simulink model "distillation"  (R2013a)
settings: Solver=ode45  StartTime=0.0  StopTime=100  RelTol=1e-3
StopFcn:
  | plot_results
libraries: simulink x4, realtime_pacer_lib x1
settings Model: Creator=tsladeche  LastModifiedBy=John
settings DataIOCC: SignalLoggingSaveFormat=ModelDataLogs
settings OptimizationCC: ExpressionDepthLimit=2147483647
settings DebuggingCC: FcnCallInpInsideContextMsg=UseLocalSettings  StrictBusMsg=Warning
settings GRTTargetCC: CombineOutputUpdateFcns=off  GRTInterface=on

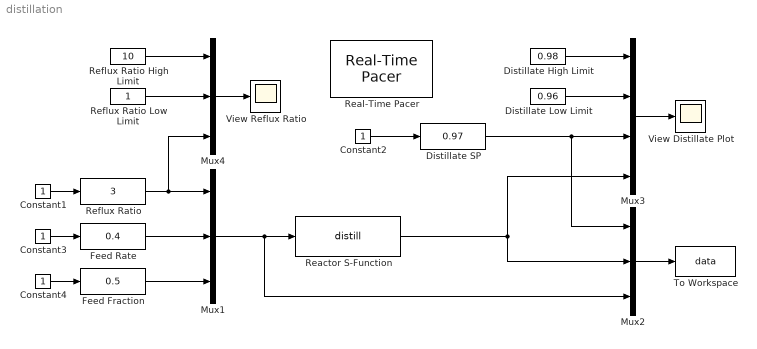
== system distillation ==
  Constant{1..4} (4 alike) : Constant
  Distillate High Limit : Constant  Value=0.98
  Distillate Low Limit : Constant  Value=0.96
  Distillate SP : simulink/Math Operations/Slider Gain  low=0.5  gain=0.97  high=1
  Feed Fraction : simulink/Math Operations/Slider Gain  low=0.1  gain=0.5  high=1
  Feed Rate : simulink/Math Operations/Slider Gain  low=0.1  gain=0.4  high=1
  Mux1 : Mux  Inputs=3
  Mux2 : Mux  Inputs=3
  Mux3 : Mux
  Mux4 : Mux  Inputs=3
  Reactor S-Function : S-Function  FunctionName=distill  EnableBusSupport=off
  Real-Time Pacer : realtime_pacer_lib/Real-Time Pacer  simTimePerRealTime=3
  Reflux Ratio : simulink/Math Operations/Slider Gain  low=1  gain=3  high=10
  Reflux Ratio High Limit : Constant  Value=10
  Reflux Ratio Low Limit : Constant
  To Workspace : ToWorkspace  VariableName=data  SampleTime=0.2  SaveFormat=Timeseries
  View Distillate Plot : Scope
      settings: ShowLegends=on  TimeRange=100  YMin=0.935  YMax=0.98  MaxDataPoints=30000
  View Reflux Ratio : Scope
      settings: ShowLegends=on  TimeRange=100  YMin=1  YMax=10  MaxDataPoints=30000
  wires:
  Mux1/1 -> Mux2/3, Reactor S-Function/1
  Constant2/1 -> Distillate SP/1
  Distillate SP/1 -> Mux2/1, Mux3/3
  Reactor S-Function/1 -> Mux3/4, Mux2/2
  Distillate High Limit/1 -> Mux3/1
  Distillate Low Limit/1 -> Mux3/2
  Mux3/1 -> View Distillate Plot/1
  Reflux Ratio/1 -> Mux4/3, Mux1/1
  Reflux Ratio High Limit/1 -> Mux4/1
  Reflux Ratio Low Limit/1 -> Mux4/2
  Mux4/1 -> View Reflux Ratio/1
  Constant1/1 -> Reflux Ratio/1
  Constant3/1 -> Feed Rate/1
  Feed Rate/1 -> Mux1/2
  Constant4/1 -> Feed Fraction/1
  Feed Fraction/1 -> Mux1/3
  Mux2/1 -> To Workspace/1
